simulink model "z7_symulacja"  (R2021a)
settings: Solver=VariableStepAuto  StartTime=0.0  StopTime=10  RelTol=1e-3
values from neighbouring files (symbols this model uses):
  L1 = - (287708*so)/3465 - (79228*so^2)/3465 - (22628*so^3)/10395 - 1168108/10395    (= 3335.19499759)    [z6i7.m]
  L2 = (79228*so)/3465 + (22628*so^2)/3465 + (6448*so^3)/10395 + 287708/10395    (= -939.456661857)    [z6i7.m]
  L3 = - (22628*so)/3465 - (6448*so^2)/3465 - (1808*so^3)/10395 - 79228/10395    (= 258.646657047)    [z6i7.m]
  sb = -8    [z4.m]    (also in z6i7.m = -5; z_dod.m = -2)
settings Model: Creator=48604  LastModifiedBy=48604

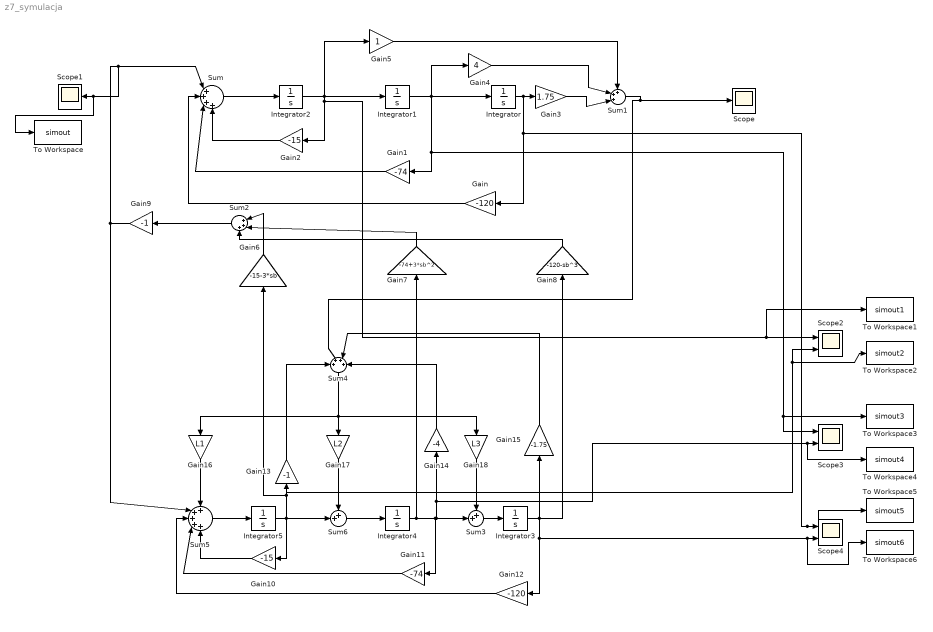
== system z7_symulacja ==
  Gain : Gain  Gain=-120
  Gain1 : Gain  Gain=-74
  Gain10 : Gain  Gain=-15
  Gain11 : Gain  Gain=-74
  Gain12 : Gain  Gain=-120
  Gain13 : Gain  Gain=-1
  Gain14 : Gain  Gain=-4
  Gain15 : Gain  Gain=-1.75
  Gain16 : Gain  Gain=L1
  Gain17 : Gain  Gain=L2
  Gain18 : Gain  Gain=L3
  Gain2 : Gain  Gain=-15
  Gain3 : Gain  Gain=1.75
  Gain4 : Gain  Gain=4
  Gain5 : Gain
  Gain6 : Gain  Gain=-15-3*sb
  Gain7 : Gain  Gain=-74+3*sb^2
  Gain8 : Gain  Gain=-120-sb^3
  Gain9 : Gain  Gain=-1
  Integrator : Integrator  InitialCondition=1
  Integrator1 : Integrator  InitialCondition=2
  Integrator2 : Integrator  InitialCondition=-1
  Integrator3 : Integrator
  Integrator4 : Integrator
  Integrator5 : Integrator
  Scope : Scope
  Scope1 : Scope
  Scope2 : Scope  NumInputPorts=2
  Scope3 : Scope  NumInputPorts=2
  Scope4 : Scope  NumInputPorts=2
  Sum : Sum  Inputs=|++++
  Sum1 : Sum  Inputs=+++|
  Sum2 : Sum  Inputs=|+++
  Sum3 : Sum  Inputs=++|
  Sum4 : Sum  Inputs=++++
  Sum5 : Sum  Inputs=+++++
  Sum6 : Sum  Inputs=++|
  To Workspace : ToWorkspace  VariableName=simout  SaveFormat=Structure With Time  SampleTime=-1
  To Workspace1 : ToWorkspace  VariableName=simout1  SaveFormat=Structure With Time  SampleTime=-1
  To Workspace2 : ToWorkspace  VariableName=simout2  SaveFormat=Structure With Time  SampleTime=-1
  To Workspace3 : ToWorkspace  VariableName=simout3  SaveFormat=Structure With Time  SampleTime=-1
  To Workspace4 : ToWorkspace  VariableName=simout4  SaveFormat=Structure With Time  SampleTime=-1
  To Workspace5 : ToWorkspace  VariableName=simout5  SaveFormat=Structure With Time  SampleTime=-1
  To Workspace6 : ToWorkspace  VariableName=simout6  SaveFormat=Structure With Time  SampleTime=-1
  wires:
  Sum4/1 -> Gain18/1, Gain17/1, Gain16/1
  Gain15/1 -> Sum4/3
  Gain18/1 -> Sum3/1
  Sum3/1 -> Integrator3/1
  Gain13/1 -> Sum4/1
  Gain10/1 -> Sum5/5
  Gain16/1 -> Sum5/1
  Sum6/1 -> Integrator4/1
  Gain14/1 -> Sum4/4
  Gain8/1 -> Sum2/3
  Gain6/1 -> Sum2/1
  Sum/1 -> Integrator2/1
  Integrator5/1 -> Gain6/1, To Workspace2/1, Scope2/2, Gain13/1, Sum6/2, Gain10/1
  Gain5/1 -> Sum1/1
  Sum1/1 -> Sum4/2, Scope/1
  Gain11/1 -> Sum5/4
  Gain1/1 -> Sum/3
  Gain2/1 -> Sum/4
  Integrator/1 -> To Workspace5/1, Scope4/1, Gain/1, Gain3/1
  Integrator1/1 -> Scope3/1, To Workspace3/1, Gain1/1, Integrator/1, Gain4/1
  Integrator3/1 -> Gain8/1, To Workspace6/1, Scope4/2, Gain12/1, Gain15/1
  Gain12/1 -> Sum5/3
  Gain3/1 -> Sum1/3
  Gain4/1 -> Sum1/2
  Gain7/1 -> Sum2/2
  Sum2/1 -> Gain9/1
  Gain9/1 -> Sum/1, To Workspace/1, Scope1/1, Sum5/2
  Integrator4/1 -> To Workspace4/1, Scope3/2, Gain14/1, Sum3/2, Gain11/1, Gain7/1
  Sum5/1 -> Integrator5/1
  Gain17/1 -> Sum6/1
  Integrator2/1 -> Integrator1/1, To Workspace1/1, Scope2/1, Gain2/1, Gain5/1
  Gain/1 -> Sum/2
